simulink model "W06_city_highway_cs"  (R2019a)
settings: Solver=ode5  StartTime=0.0  StopTime=inf  FixedStep=1/60  RelTol=1e-3
PreLoadFcn:
  | mbxruntime.callbacks.PreLoadFcn(bdroot);
PostLoadFcn:
  | mbxruntime.callbacks.PostLoadFcn(bdroot);
InitFcn:
  | mbxruntime.callbacks.InitFcn(bdroot);
StartFcn:
  | mbxruntime.callbacks.StartFcn(bdroot);
StopFcn:
  | mbxruntime.callbacks.StopFcn(bdroot);
model workspace: external: MAT-File .\W06_city_highway_cs_hws.mat (data not in the file)
undefined symbols (not defined in the file or in its folder): DiscIntNeverNeededParam, FovAzimuth, FovAzimuthDefined, FovElevation, FovElevationDefined, Header, InitImageOutputDir, LocationX, LocationXDefined, LocationY, LocationYDefined, LocationZ, LocationZDefined, Orientation, OrientationPitch, OrientationPitchDefined, OrientationRoll, OrientationRollDefined, OrientationYaw, OrientationYawDefined, Poses, Poses_SL_Info, Position, W06_city_highway_cs_0270c22595f3b0e3, W06_city_highway_cs_086892688dd32ddc, W06_city_highway_cs_328c49ac39fca66b, W06_city_highway_cs_35ce05381b8ebe8c, W06_city_highway_cs_47b384f162638175, W06_city_highway_cs_766f76ce4de94dd5, W06_city_highway_cs_8c547f67cb81ffba, W06_city_highway_cs_aed52f2a7724a4f9, W06_city_highway_cs_Audi_A8_Sedan_1_Path_pathUniqueID, W06_city_highway_cs_b74cbb1f9f7331b5, W06_city_highway_cs_Citroen_C3_Hatchback_1_Path_pathUniqueID, W06_city_highway_cs_d395f8835e0c28b3, W06_city_highway_cs_e5f9d1759e19e2b4, W06_city_highway_cs_Toyota_Previa_MPV_1_Path_pathUniqueID
libraries: adeye_lib x26, simulink_extras x24, robotlib x7, sharedtransform x4, PreScanSimulinkLibrary x2, PreScanUsefulBlocks x1
(part 6 of 8)

== system W06_city_highway_cs/RoadsideLight_NL_2/Red_Mux ==
  MSCD [Cd] : Inport
  Position (xyz) [m] : Inport  Port=2
  Orientation (RPY) [deg] : Inport  Port=3
  Color [-] : Inport  Port=4
  TextureResourceID [-] : Inport  Port=5
  Bus Creator : BusCreator  Inputs='Intensity','Position','Orientation','Color','TextureResourceID'  OutDataTypeStr=Bus: PRESCAN_VISULIGHTACTUATOR_DATA  NonVirtualBus=on
  Bus Creator1 : BusCreator  Inputs=3  OutDataTypeStr=Bus: PRESCAN_RGB_DATA  NonVirtualBus=on
  Bus Creator2 : BusCreator  Inputs=3  OutDataTypeStr=Bus: PRESCAN_RPY_DATA  NonVirtualBus=on
  Bus Creator3 : BusCreator  Inputs=3  OutDataTypeStr=Bus: PRESCAN_XYZ_DATA  NonVirtualBus=on
  Data Type Conversion : DataTypeConversion  OutDataTypeStr=int32  RndMeth=Nearest
  Degrees to Radians : simulink_extras/Transformations/Degrees to Radians
  Demux : Demux  Outputs=3
  Demux1 : Demux  Outputs=3
  Demux2 : Demux  Outputs=3
  Lights : Outport
  wires:
  TextureResourceID [-]/1 -> Data Type Conversion/1  "TextureResourceID"
  MSCD [Cd]/1 -> Bus Creator/1  "Intensity"
  Bus Creator/1 -> Lights/1
  Demux/1 -> Bus Creator1/1  "R"
  Demux/2 -> Bus Creator1/2  "G"
  Demux/3 -> Bus Creator1/3  "B"
  Color [-]/1 -> Demux/1  "Color"
  Bus Creator1/1 -> Bus Creator/4  "Color"
  Demux1/1 -> Bus Creator2/1  "Roll"
  Demux1/2 -> Bus Creator2/2  "Pitch"
  Demux1/3 -> Bus Creator2/3  "Yaw"
  Orientation (RPY) [deg]/1 -> Degrees to Radians/1  "Orientation"
  Bus Creator2/1 -> Bus Creator/3  "Orientation"
  Demux2/1 -> Bus Creator3/1  "X"
  Demux2/2 -> Bus Creator3/2  "Y"
  Demux2/3 -> Bus Creator3/3  "Z"
  Position (xyz) [m]/1 -> Demux2/1  "Position"
  Bus Creator3/1 -> Bus Creator/2  "Position"
  Data Type Conversion/1 -> Bus Creator/5  "TextureResourceID"
  Degrees to Radians/1 -> Demux1/1

== system W06_city_highway_cs/RoadsideLight_NL_3/Green_Mux ==
  MSCD [Cd] : Inport
  Position (xyz) [m] : Inport  Port=2
  Orientation (RPY) [deg] : Inport  Port=3
  Color [-] : Inport  Port=4
  TextureResourceID [-] : Inport  Port=5
  Bus Creator : BusCreator  Inputs='Intensity','Position','Orientation','Color','TextureResourceID'  OutDataTypeStr=Bus: PRESCAN_VISULIGHTACTUATOR_DATA  NonVirtualBus=on
  Bus Creator1 : BusCreator  Inputs=3  OutDataTypeStr=Bus: PRESCAN_RGB_DATA  NonVirtualBus=on
  Bus Creator2 : BusCreator  Inputs=3  OutDataTypeStr=Bus: PRESCAN_RPY_DATA  NonVirtualBus=on
  Bus Creator3 : BusCreator  Inputs=3  OutDataTypeStr=Bus: PRESCAN_XYZ_DATA  NonVirtualBus=on
  Data Type Conversion : DataTypeConversion  OutDataTypeStr=int32  RndMeth=Nearest
  Degrees to Radians : simulink_extras/Transformations/Degrees to Radians
  Demux : Demux  Outputs=3
  Demux1 : Demux  Outputs=3
  Demux2 : Demux  Outputs=3
  Lights : Outport
  wires:
  TextureResourceID [-]/1 -> Data Type Conversion/1  "TextureResourceID"
  MSCD [Cd]/1 -> Bus Creator/1  "Intensity"
  Bus Creator/1 -> Lights/1
  Demux/1 -> Bus Creator1/1  "R"
  Demux/2 -> Bus Creator1/2  "G"
  Demux/3 -> Bus Creator1/3  "B"
  Color [-]/1 -> Demux/1  "Color"
  Bus Creator1/1 -> Bus Creator/4  "Color"
  Demux1/1 -> Bus Creator2/1  "Roll"
  Demux1/2 -> Bus Creator2/2  "Pitch"
  Demux1/3 -> Bus Creator2/3  "Yaw"
  Orientation (RPY) [deg]/1 -> Degrees to Radians/1  "Orientation"
  Bus Creator2/1 -> Bus Creator/3  "Orientation"
  Demux2/1 -> Bus Creator3/1  "X"
  Demux2/2 -> Bus Creator3/2  "Y"
  Demux2/3 -> Bus Creator3/3  "Z"
  Position (xyz) [m]/1 -> Demux2/1  "Position"
  Bus Creator3/1 -> Bus Creator/2  "Position"
  Data Type Conversion/1 -> Bus Creator/5  "TextureResourceID"
  Degrees to Radians/1 -> Demux1/1

== system W06_city_highway_cs/RoadsideLight_NL_3/Orange_Mux ==
  MSCD [Cd] : Inport
  Position (xyz) [m] : Inport  Port=2
  Orientation (RPY) [deg] : Inport  Port=3
  Color [-] : Inport  Port=4
  TextureResourceID [-] : Inport  Port=5
  Bus Creator : BusCreator  Inputs='Intensity','Position','Orientation','Color','TextureResourceID'  OutDataTypeStr=Bus: PRESCAN_VISULIGHTACTUATOR_DATA  NonVirtualBus=on
  Bus Creator1 : BusCreator  Inputs=3  OutDataTypeStr=Bus: PRESCAN_RGB_DATA  NonVirtualBus=on
  Bus Creator2 : BusCreator  Inputs=3  OutDataTypeStr=Bus: PRESCAN_RPY_DATA  NonVirtualBus=on
  Bus Creator3 : BusCreator  Inputs=3  OutDataTypeStr=Bus: PRESCAN_XYZ_DATA  NonVirtualBus=on
  Data Type Conversion : DataTypeConversion  OutDataTypeStr=int32  RndMeth=Nearest
  Degrees to Radians : simulink_extras/Transformations/Degrees to Radians
  Demux : Demux  Outputs=3
  Demux1 : Demux  Outputs=3
  Demux2 : Demux  Outputs=3
  Lights : Outport
  wires:
  TextureResourceID [-]/1 -> Data Type Conversion/1  "TextureResourceID"
  MSCD [Cd]/1 -> Bus Creator/1  "Intensity"
  Bus Creator/1 -> Lights/1
  Demux/1 -> Bus Creator1/1  "R"
  Demux/2 -> Bus Creator1/2  "G"
  Demux/3 -> Bus Creator1/3  "B"
  Color [-]/1 -> Demux/1  "Color"
  Bus Creator1/1 -> Bus Creator/4  "Color"
  Demux1/1 -> Bus Creator2/1  "Roll"
  Demux1/2 -> Bus Creator2/2  "Pitch"
  Demux1/3 -> Bus Creator2/3  "Yaw"
  Orientation (RPY) [deg]/1 -> Degrees to Radians/1  "Orientation"
  Bus Creator2/1 -> Bus Creator/3  "Orientation"
  Demux2/1 -> Bus Creator3/1  "X"
  Demux2/2 -> Bus Creator3/2  "Y"
  Demux2/3 -> Bus Creator3/3  "Z"
  Position (xyz) [m]/1 -> Demux2/1  "Position"
  Bus Creator3/1 -> Bus Creator/2  "Position"
  Data Type Conversion/1 -> Bus Creator/5  "TextureResourceID"
  Degrees to Radians/1 -> Demux1/1

== system W06_city_highway_cs/RoadsideLight_NL_3/Red_Mux ==
  MSCD [Cd] : Inport
  Position (xyz) [m] : Inport  Port=2
  Orientation (RPY) [deg] : Inport  Port=3
  Color [-] : Inport  Port=4
  TextureResourceID [-] : Inport  Port=5
  Bus Creator : BusCreator  Inputs='Intensity','Position','Orientation','Color','TextureResourceID'  OutDataTypeStr=Bus: PRESCAN_VISULIGHTACTUATOR_DATA  NonVirtualBus=on
  Bus Creator1 : BusCreator  Inputs=3  OutDataTypeStr=Bus: PRESCAN_RGB_DATA  NonVirtualBus=on
  Bus Creator2 : BusCreator  Inputs=3  OutDataTypeStr=Bus: PRESCAN_RPY_DATA  NonVirtualBus=on
  Bus Creator3 : BusCreator  Inputs=3  OutDataTypeStr=Bus: PRESCAN_XYZ_DATA  NonVirtualBus=on
  Data Type Conversion : DataTypeConversion  OutDataTypeStr=int32  RndMeth=Nearest
  Degrees to Radians : simulink_extras/Transformations/Degrees to Radians
  Demux : Demux  Outputs=3
  Demux1 : Demux  Outputs=3
  Demux2 : Demux  Outputs=3
  Lights : Outport
  wires:
  TextureResourceID [-]/1 -> Data Type Conversion/1  "TextureResourceID"
  MSCD [Cd]/1 -> Bus Creator/1  "Intensity"
  Bus Creator/1 -> Lights/1
  Demux/1 -> Bus Creator1/1  "R"
  Demux/2 -> Bus Creator1/2  "G"
  Demux/3 -> Bus Creator1/3  "B"
  Color [-]/1 -> Demux/1  "Color"
  Bus Creator1/1 -> Bus Creator/4  "Color"
  Demux1/1 -> Bus Creator2/1  "Roll"
  Demux1/2 -> Bus Creator2/2  "Pitch"
  Demux1/3 -> Bus Creator2/3  "Yaw"
  Orientation (RPY) [deg]/1 -> Degrees to Radians/1  "Orientation"
  Bus Creator2/1 -> Bus Creator/3  "Orientation"
  Demux2/1 -> Bus Creator3/1  "X"
  Demux2/2 -> Bus Creator3/2  "Y"
  Demux2/3 -> Bus Creator3/3  "Z"
  Position (xyz) [m]/1 -> Demux2/1  "Position"
  Bus Creator3/1 -> Bus Creator/2  "Position"
  Data Type Conversion/1 -> Bus Creator/5  "TextureResourceID"
  Degrees to Radians/1 -> Demux1/1

== system W06_city_highway_cs/RoadsideLight_NL_4/Green_Mux ==
  MSCD [Cd] : Inport
  Position (xyz) [m] : Inport  Port=2
  Orientation (RPY) [deg] : Inport  Port=3
  Color [-] : Inport  Port=4
  TextureResourceID [-] : Inport  Port=5
  Bus Creator : BusCreator  Inputs='Intensity','Position','Orientation','Color','TextureResourceID'  OutDataTypeStr=Bus: PRESCAN_VISULIGHTACTUATOR_DATA  NonVirtualBus=on
  Bus Creator1 : BusCreator  Inputs=3  OutDataTypeStr=Bus: PRESCAN_RGB_DATA  NonVirtualBus=on
  Bus Creator2 : BusCreator  Inputs=3  OutDataTypeStr=Bus: PRESCAN_RPY_DATA  NonVirtualBus=on
  Bus Creator3 : BusCreator  Inputs=3  OutDataTypeStr=Bus: PRESCAN_XYZ_DATA  NonVirtualBus=on
  Data Type Conversion : DataTypeConversion  OutDataTypeStr=int32  RndMeth=Nearest
  Degrees to Radians : simulink_extras/Transformations/Degrees to Radians
  Demux : Demux  Outputs=3
  Demux1 : Demux  Outputs=3
  Demux2 : Demux  Outputs=3
  Lights : Outport
  wires:
  TextureResourceID [-]/1 -> Data Type Conversion/1  "TextureResourceID"
  MSCD [Cd]/1 -> Bus Creator/1  "Intensity"
  Bus Creator/1 -> Lights/1
  Demux/1 -> Bus Creator1/1  "R"
  Demux/2 -> Bus Creator1/2  "G"
  Demux/3 -> Bus Creator1/3  "B"
  Color [-]/1 -> Demux/1  "Color"
  Bus Creator1/1 -> Bus Creator/4  "Color"
  Demux1/1 -> Bus Creator2/1  "Roll"
  Demux1/2 -> Bus Creator2/2  "Pitch"
  Demux1/3 -> Bus Creator2/3  "Yaw"
  Orientation (RPY) [deg]/1 -> Degrees to Radians/1  "Orientation"
  Bus Creator2/1 -> Bus Creator/3  "Orientation"
  Demux2/1 -> Bus Creator3/1  "X"
  Demux2/2 -> Bus Creator3/2  "Y"
  Demux2/3 -> Bus Creator3/3  "Z"
  Position (xyz) [m]/1 -> Demux2/1  "Position"
  Bus Creator3/1 -> Bus Creator/2  "Position"
  Data Type Conversion/1 -> Bus Creator/5  "TextureResourceID"
  Degrees to Radians/1 -> Demux1/1

== system W06_city_highway_cs/RoadsideLight_NL_4/Orange_Mux ==
  MSCD [Cd] : Inport
  Position (xyz) [m] : Inport  Port=2
  Orientation (RPY) [deg] : Inport  Port=3
  Color [-] : Inport  Port=4
  TextureResourceID [-] : Inport  Port=5
  Bus Creator : BusCreator  Inputs='Intensity','Position','Orientation','Color','TextureResourceID'  OutDataTypeStr=Bus: PRESCAN_VISULIGHTACTUATOR_DATA  NonVirtualBus=on
  Bus Creator1 : BusCreator  Inputs=3  OutDataTypeStr=Bus: PRESCAN_RGB_DATA  NonVirtualBus=on
  Bus Creator2 : BusCreator  Inputs=3  OutDataTypeStr=Bus: PRESCAN_RPY_DATA  NonVirtualBus=on
  Bus Creator3 : BusCreator  Inputs=3  OutDataTypeStr=Bus: PRESCAN_XYZ_DATA  NonVirtualBus=on
  Data Type Conversion : DataTypeConversion  OutDataTypeStr=int32  RndMeth=Nearest
  Degrees to Radians : simulink_extras/Transformations/Degrees to Radians
  Demux : Demux  Outputs=3
  Demux1 : Demux  Outputs=3
  Demux2 : Demux  Outputs=3
  Lights : Outport
  wires:
  TextureResourceID [-]/1 -> Data Type Conversion/1  "TextureResourceID"
  MSCD [Cd]/1 -> Bus Creator/1  "Intensity"
  Bus Creator/1 -> Lights/1
  Demux/1 -> Bus Creator1/1  "R"
  Demux/2 -> Bus Creator1/2  "G"
  Demux/3 -> Bus Creator1/3  "B"
  Color [-]/1 -> Demux/1  "Color"
  Bus Creator1/1 -> Bus Creator/4  "Color"
  Demux1/1 -> Bus Creator2/1  "Roll"
  Demux1/2 -> Bus Creator2/2  "Pitch"
  Demux1/3 -> Bus Creator2/3  "Yaw"
  Orientation (RPY) [deg]/1 -> Degrees to Radians/1  "Orientation"
  Bus Creator2/1 -> Bus Creator/3  "Orientation"
  Demux2/1 -> Bus Creator3/1  "X"
  Demux2/2 -> Bus Creator3/2  "Y"
  Demux2/3 -> Bus Creator3/3  "Z"
  Position (xyz) [m]/1 -> Demux2/1  "Position"
  Bus Creator3/1 -> Bus Creator/2  "Position"
  Data Type Conversion/1 -> Bus Creator/5  "TextureResourceID"
  Degrees to Radians/1 -> Demux1/1

== system W06_city_highway_cs/RoadsideLight_NL_4/Red_Mux ==
  MSCD [Cd] : Inport
  Position (xyz) [m] : Inport  Port=2
  Orientation (RPY) [deg] : Inport  Port=3
  Color [-] : Inport  Port=4
  TextureResourceID [-] : Inport  Port=5
  Bus Creator : BusCreator  Inputs='Intensity','Position','Orientation','Color','TextureResourceID'  OutDataTypeStr=Bus: PRESCAN_VISULIGHTACTUATOR_DATA  NonVirtualBus=on
  Bus Creator1 : BusCreator  Inputs=3  OutDataTypeStr=Bus: PRESCAN_RGB_DATA  NonVirtualBus=on
  Bus Creator2 : BusCreator  Inputs=3  OutDataTypeStr=Bus: PRESCAN_RPY_DATA  NonVirtualBus=on
  Bus Creator3 : BusCreator  Inputs=3  OutDataTypeStr=Bus: PRESCAN_XYZ_DATA  NonVirtualBus=on
  Data Type Conversion : DataTypeConversion  OutDataTypeStr=int32  RndMeth=Nearest
  Degrees to Radians : simulink_extras/Transformations/Degrees to Radians
  Demux : Demux  Outputs=3
  Demux1 : Demux  Outputs=3
  Demux2 : Demux  Outputs=3
  Lights : Outport
  wires:
  TextureResourceID [-]/1 -> Data Type Conversion/1  "TextureResourceID"
  MSCD [Cd]/1 -> Bus Creator/1  "Intensity"
  Bus Creator/1 -> Lights/1
  Demux/1 -> Bus Creator1/1  "R"
  Demux/2 -> Bus Creator1/2  "G"
  Demux/3 -> Bus Creator1/3  "B"
  Color [-]/1 -> Demux/1  "Color"
  Bus Creator1/1 -> Bus Creator/4  "Color"
  Demux1/1 -> Bus Creator2/1  "Roll"
  Demux1/2 -> Bus Creator2/2  "Pitch"
  Demux1/3 -> Bus Creator2/3  "Yaw"
  Orientation (RPY) [deg]/1 -> Degrees to Radians/1  "Orientation"
  Bus Creator2/1 -> Bus Creator/3  "Orientation"
  Demux2/1 -> Bus Creator3/1  "X"
  Demux2/2 -> Bus Creator3/2  "Y"
  Demux2/3 -> Bus Creator3/3  "Z"
  Position (xyz) [m]/1 -> Demux2/1  "Position"
  Bus Creator3/1 -> Bus Creator/2  "Position"
  Data Type Conversion/1 -> Bus Creator/5  "TextureResourceID"
  Degrees to Radians/1 -> Demux1/1

== system W06_city_highway_cs/Toyota_Previa_MPV_1/Car_Pos_and_Orient ==
  In1 : Inport
  In2 : Inport  Port=2
  In3 : Inport  Port=3
  In4 : Inport  Port=4
  In5 : Inport  Port=5
  In6 : Inport  Port=6
  Data Type Conversion : DataTypeConversion
  Data Type Conversion1 : DataTypeConversion
  Data Type Conversion2 : DataTypeConversion
  Degrees to Radians1 : simulink_extras/Transformations/Degrees to Radians
  Degrees to Radians2 : simulink_extras/Transformations/Degrees to Radians
  Degrees to Radians5 : simulink_extras/Transformations/Degrees to Radians
  Mux : Mux
  Rotation Angles to Quaternions : sharedtransform/Rotation Angles to Quaternions  rotationOrder=XYZ  aMode=aMode
      settings: SourceProductName=Aerospace Blockset  SourceProductBaseCode=AE
  Vector Concatenate2 : Concatenate  NumInputs=3
  Out1 : Outport
  wires:
  Degrees to Radians1/1 -> Vector Concatenate2/2
  Degrees to Radians5/1 -> Vector Concatenate2/1
  Vector Concatenate2/1 -> Rotation Angles to Quaternions/1
  Degrees to Radians2/1 -> Vector Concatenate2/3
  In1/1 -> Data Type Conversion/1
  In2/1 -> Data Type Conversion1/1
  In3/1 -> Data Type Conversion2/1
  In4/1 -> Degrees to Radians5/1
  In5/1 -> Degrees to Radians1/1
  In6/1 -> Degrees to Radians2/1
  Data Type Conversion/1 -> Mux/1
  Data Type Conversion1/1 -> Mux/2
  Data Type Conversion2/1 -> Mux/3
  Rotation Angles to Quaternions/1 -> Mux/4
  Mux/1 -> Out1/1

== system W06_city_highway_cs/Toyota_Previa_MPV_1/SELF_Demux ==
  SELF : Inport  OutDataTypeStr=Bus: PRESCAN_SELFSENSORDATA
  Bus Selector : BusSelector  OutputSignals=PositionX,PositionY,PositionZ,OrientationRoll,OrientationPitch,OrientationYaw,Velocity,Yaw_rate,Lat,Long,Alt
  Demux2 : Demux  Outputs=3
  Gain : Gain  Gain=180/pi
  Gain1 : Gain  Gain=180/pi
  Vector Concatenate1 : Concatenate  NumInputs=3
  compas converter : Subsystem
  x [m] : Outport
  y [m] : Outport  Port=2
  z [m] : Outport  Port=3
  rotx [deg] : Outport  Port=4
  roty [deg] : Outport  Port=5
  rotz [deg] : Outport  Port=6
  GPS lat [deg] : Outport  Port=7
  GPS long [deg] : Outport  Port=8
  GPS alt [m] : Outport  Port=9
  velocity [m/s] : Outport  Port=10
  heading [deg] : Outport  Port=11
  yaw rate [deg/s] : Outport  Port=12
  wires:
  Bus Selector/11 -> GPS alt [m]/1  "<Alt>"
  Bus Selector/10 -> GPS long [deg]/1  "<Long>"
  Bus Selector/9 -> GPS lat [deg]/1  "<Lat>"
  Bus Selector/8 -> Gain1/1  "<Yaw_rate>"
  Bus Selector/7 -> velocity [m/s]/1  "<Velocity>"
  Bus Selector/6 -> compas converter/1(rotz [rad]), Vector Concatenate1/3  "<OrientationYaw>"
  Bus Selector/5 -> Vector Concatenate1/2  "<OrientationPitch>"
  Bus Selector/4 -> Vector Concatenate1/1  "<OrientationRoll>"
  Vector Concatenate1/1 -> Gain/1
  Bus Selector/3 -> z [m]/1  "<PositionZ>"
  Bus Selector/2 -> y [m]/1  "<PositionY>"
  Bus Selector/1 -> x [m]/1  "<PositionX>"
  SELF/1 -> Bus Selector/1
  Gain/1 -> Demux2/1
  Demux2/1 -> rotx [deg]/1
  Demux2/2 -> roty [deg]/1
  Demux2/3 -> rotz [deg]/1
  compas converter/1(heading [deg]) -> heading [deg]/1
  Gain1/1 -> yaw rate [deg/s]/1

== system W06_city_highway_cs/Toyota_Previa_MPV_1/message_creator ==
  In1 : Inport
  Blank Message4 : robotlib/Blank Message  messageClass=Message  entityType=geometry_msgs/Pose  messageType=geometry_msgs/Pose  SampleTime=inf
      settings: SourceProductBaseCode=RO
  Bus Assignment3 : BusAssignment  AssignedSignals=Position.X,Position.Y,Position.Z,Orientation.W,Orientation.X,Orientation.Y,Orientation.Z
  Demux : Demux  Outputs=7
  Out1 : Outport
  wires:
  Blank Message4/1 -> Bus Assignment3/1
  Demux/4 -> Bus Assignment3/5
  Demux/3 -> Bus Assignment3/4
  Demux/5 -> Bus Assignment3/6
  Demux/7 -> Bus Assignment3/8
  Demux/2 -> Bus Assignment3/3
  In1/1 -> Demux/1
  Demux/6 -> Bus Assignment3/7
  Demux/1 -> Bus Assignment3/2
  Bus Assignment3/1 -> Out1/1

== system W06_city_highway_cs/Audi_A8_Sedan_1/SELF_Demux/compas converter ==
  rotz [rad] : Inport
  cart2compas : Subsystem
  rad2deg : Gain  Gain=180/pi
  heading [deg] : Outport
  wires:
  rad2deg/1 -> cart2compas/1(Angle [deg])
  rotz [rad]/1 -> rad2deg/1
  cart2compas/1(heading [deg]) -> heading [deg]/1

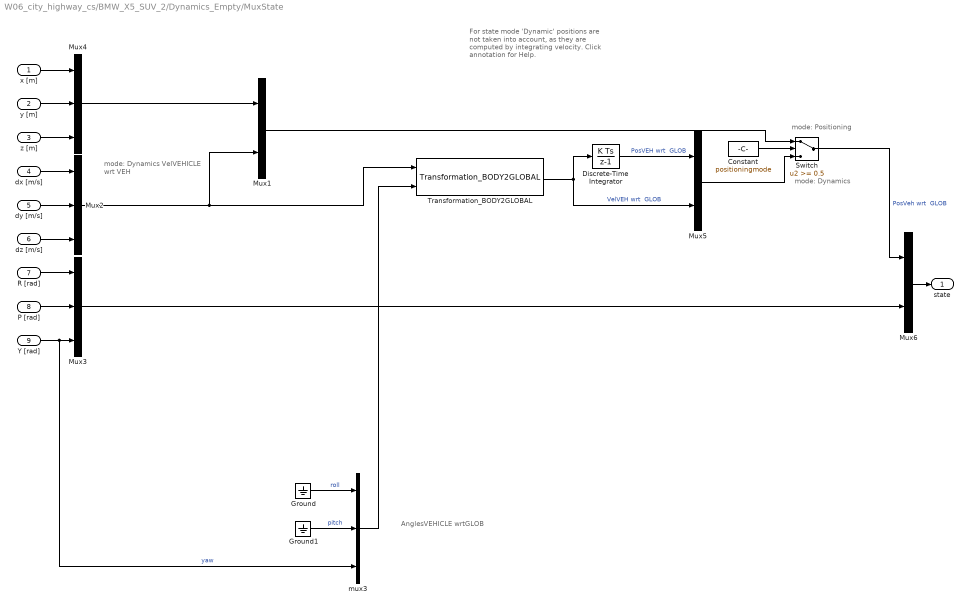
== system W06_city_highway_cs/BMW_X5_SUV_2/Dynamics_Empty/MuxState ==
  note: mode: Dynamics
  note: mode: Positioning
  note: mode: Dynamics
      | VelVEHICLE
      | wrt VEH
  note: AnglesVEHICLE
      | wrtGLOB
  note: For state mode 'Dynamic' positions
      | are not taken into account, as they
      | are computed by integrating velocity.
      | Click annotation for Help.
  x [m] : Inport  SampleTime=TimeStep
  y [m] : Inport  Port=2  SampleTime=TimeStep
  z [m] : Inport  Port=3  SampleTime=TimeStep
  dx [m/s] : Inport  Port=4  SampleTime=TimeStep
  dy [m/s] : Inport  Port=5  SampleTime=TimeStep
  dz [m/s] : Inport  Port=6  SampleTime=TimeStep
  R [rad] : Inport  Port=7  SampleTime=TimeStep
  P [rad] : Inport  Port=8  SampleTime=TimeStep
  Y [rad] : Inport  Port=9  SampleTime=TimeStep
  Constant : Constant  DisableCoverage=on  Value=positioningmode
  Discrete-Time Integrator : DiscreteIntegrator  SampleTime=TimeStep  ICPrevOutput=DiscIntNeverNeededParam  ICPrevScaledInput=DiscIntNeverNeededParam
  Ground : Ground
  Ground1 : Ground
  Mux1 : Mux  Inputs=[3 3]
  Mux2 : Mux  Inputs=3
  Mux3 : Mux  Inputs=3
  Mux4 : Mux  Inputs=3
  Mux5 : Mux  Inputs=[3 3]
  Mux6 : Mux  Inputs=[6 3]
  Switch : Switch  Threshold=0.5
  Transformation_BODY2GLOBAL : PreScanSimulinkLibrary/Simple_Vehicle_Dynamics/Chassis/MuxDynState/Transformation_BODY2GLOBAL  SystemSampleTime=-1
  mux3 : Mux  Inputs=3
  state : Outport
  wires:
  Constant/1 -> Switch/2
  Mux6/1 -> state/1
  Mux4/1 -> Mux1/1
  Mux5/1 -> Switch/3
  Mux1/1 -> Switch/1
  Switch/1 -> Mux6/1  "PosVeh wrt  GLOB"
  P [rad]/1 -> Mux3/2
  R [rad]/1 -> Mux3/1
  dz [m/s]/1 -> Mux2/3
  dy [m/s]/1 -> Mux2/2
  dx [m/s]/1 -> Mux2/1
  z [m]/1 -> Mux4/3
  y [m]/1 -> Mux4/2
  x [m]/1 -> Mux4/1
  Ground1/1 -> mux3/2  "pitch"
  Y [rad]/1 -> mux3/3, Mux3/3  "yaw"
  Mux3/1 -> Mux6/2
  Transformation_BODY2GLOBAL/1 -> Discrete-Time Integrator/1, Mux5/2  "VelVEH wrt  GLOB"
  mux3/1 -> Transformation_BODY2GLOBAL/2
  Ground/1 -> mux3/1  "roll"
  Mux2/1 -> Mux1/2, Transformation_BODY2GLOBAL/1
  Discrete-Time Integrator/1 -> Mux5/1  "PosVEH wrt  GLOB"

== system W06_city_highway_cs/BMW_X5_SUV_2/Dynamics_Empty/STATE_BMW_X5_SUV_2 ==
  State : Inport  SampleTime=TimeStep
  Bus Creator : BusCreator  Inputs=15  OutDataTypeStr=Bus: PRESCAN_STATEACTUATORDATA  NonVirtualBus=on
  Constant : Constant  Value=0
  Demux : Demux  Outputs=15
  Mux : Mux  Inputs=3
  Mux1 : Mux  Inputs=3
  Mux2 : Mux  Inputs=3
  iniBODYAngles wrtVEH [rad] : Constant  Value=Roll0  SampleTime=TimeStep
  iniBODYAngles wrtVEH [rad]1 : Constant  Value=Pitch0  SampleTime=TimeStep
  iniVEHAngles wrtGLOB [rad] : Constant  Value=Yaw0  SampleTime=TimeStep
  iniVEHposition wrtGLOB [m] : Constant  Value=x0  SampleTime=TimeStep
  iniVEHposition wrtGLOB [m]1 : Constant  Value=y0  SampleTime=TimeStep
  iniVEHposition wrtGLOB [m]2 : Constant  Value=z0  SampleTime=TimeStep
  state2FullState : PreScanSimulinkLibrary/state2FullState  SystemSampleTime=-1
  StateBus : Outport  OutDataTypeStr=Bus: PRESCAN_STATEACTUATORDATA
  wires:
  Mux2/1 -> state2FullState/4
  iniVEHAngles wrtGLOB [rad]/1 -> Mux2/3
  Mux1/1 -> state2FullState/3
  Constant/1 -> Mux2/1, Mux2/2, Mux1/3
  iniBODYAngles wrtVEH [rad]1/1 -> Mux1/2
  iniBODYAngles wrtVEH [rad]/1 -> Mux1/1
  Mux/1 -> state2FullState/2
  iniVEHposition wrtGLOB [m]2/1 -> Mux/3
  iniVEHposition wrtGLOB [m]/1 -> Mux/1
  iniVEHposition wrtGLOB [m]1/1 -> Mux/2
  Demux/15 -> Bus Creator/15  "AngularVelocityYaw"
  Demux/14 -> Bus Creator/14  "AngularVelocityPitch"
  Demux/13 -> Bus Creator/13  "AngularVelocityRoll"
  Demux/12 -> Bus Creator/12  "OrientationYaw"
  Demux/11 -> Bus Creator/11  "OrientationPitch"
  Demux/10 -> Bus Creator/10  "OrientationRoll"
  Demux/9 -> Bus Creator/9  "AccelerationZ"
  Demux/8 -> Bus Creator/8  "AccelerationY"
  Demux/7 -> Bus Creator/7  "AccelerationX"
  Demux/6 -> Bus Creator/6  "VelocityZ"
  Demux/5 -> Bus Creator/5  "VelocityY"
  Demux/4 -> Bus Creator/4  "VelocityX"
  Demux/3 -> Bus Creator/3  "PositionZ"
  Demux/2 -> Bus Creator/2  "PositionY"
  Demux/1 -> Bus Creator/1  "PositionX"
  state2FullState/1 -> Demux/1
  State/1 -> state2FullState/1
  Bus Creator/1 -> StateBus/1

== system W06_city_highway_cs/BMW_X5_SUV_2/Dynamics_Empty/Subsystem ==
  note: Current
  note: Desired
  In1 : Inport
  In2 : Inport  Port=2
  Constant : Constant  Value=0.05
  If : If  NumInputs=2  IfExpression=u1 > u2  ElseIfExpressions=u1 > -u2
  If Action Subsystem : Subsystem  TreatAsAtomicUnit=on
  If Action Subsystem1 : Subsystem  TreatAsAtomicUnit=on
  If Action Subsystem2 : Subsystem  TreatAsAtomicUnit=on
  Merge : Merge  Inputs=3
  Subtract : Sum  Inputs=-+
  Out1 : Outport
  wires:
  Constant/1 -> If/2, If Action Subsystem/2(In2), If Action Subsystem1/2(In2)
  Subtract/1 -> If/1
  In2/1 -> If Action Subsystem2/1(In1), Subtract/2
  In1/1 -> Subtract/1, If Action Subsystem/1(In1), If Action Subsystem1/1(In1)
  If Action Subsystem1/1(Out1) -> Merge/3
  If/1 -> If Action Subsystem/Action
  If/2 -> If Action Subsystem2/Action
  If Action Subsystem2/1(Out1) -> Merge/2
  Merge/1 -> Out1/1
  If/3 -> If Action Subsystem1/Action
  If Action Subsystem/1(Out1) -> Merge/1

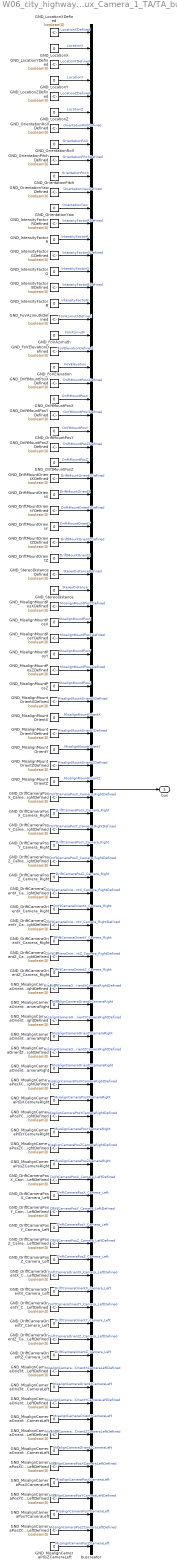
== system W06_city_highway_cs/BMW_X5_SUV_2/Mux_Camera_1_TA/TA_bus ==
  GND_DriftCameraOrientX_Camera_Left : Constant  Value=0
  GND_DriftCameraOrientX_Camera_LeftDefined : Constant  Value=boolean(0)
  GND_DriftCameraOrientX_Camera_Right : Constant  Value=0
  GND_DriftCameraOrientX_Camera_RightDefined : Constant  Value=boolean(0)
  GND_DriftCameraOrientY_Camera_Left : Constant  Value=0
  GND_DriftCameraOrientY_Camera_LeftDefined : Constant  Value=boolean(0)
  GND_DriftCameraOrientY_Camera_Right : Constant  Value=0
  GND_DriftCameraOrientY_Camera_RightDefined : Constant  Value=boolean(0)
  GND_DriftCameraOrientZ_Camera_Left : Constant  Value=0
  GND_DriftCameraOrientZ_Camera_LeftDefined : Constant  Value=boolean(0)
  GND_DriftCameraOrientZ_Camera_Right : Constant  Value=0
  GND_DriftCameraOrientZ_Camera_RightDefined : Constant  Value=boolean(0)
  GND_DriftCameraPosX_Camera_Left : Constant  Value=0
  GND_DriftCameraPosX_Camera_LeftDefined : Constant  Value=boolean(0)
  GND_DriftCameraPosX_Camera_Right : Constant  Value=0
  GND_DriftCameraPosX_Camera_RightDefined : Constant  Value=boolean(0)
  GND_DriftCameraPosY_Camera_Left : Constant  Value=0
  GND_DriftCameraPosY_Camera_LeftDefined : Constant  Value=boolean(0)
  GND_DriftCameraPosY_Camera_Right : Constant  Value=0
  GND_DriftCameraPosY_Camera_RightDefined : Constant  Value=boolean(0)
  GND_DriftCameraPosZ_Camera_Left : Constant  Value=0
  GND_DriftCameraPosZ_Camera_LeftDefined : Constant  Value=boolean(0)
  GND_DriftCameraPosZ_Camera_Right : Constant  Value=0
  GND_DriftCameraPosZ_Camera_RightDefined : Constant  Value=boolean(0)
  GND_DriftMountOrientX : Constant  Value=0
  GND_DriftMountOrientXDefined : Constant  Value=boolean(0)
  GND_DriftMountOrientY : Constant  Value=0
  GND_DriftMountOrientYDefined : Constant  Value=boolean(0)
  GND_DriftMountOrientZ : Constant  Value=0
  GND_DriftMountOrientZDefined : Constant  Value=boolean(0)
  GND_DriftMountPosX : Constant  Value=0
  GND_DriftMountPosXDefined : Constant  Value=boolean(0)
  GND_DriftMountPosY : Constant  Value=0
  GND_DriftMountPosYDefined : Constant  Value=boolean(0)
  GND_DriftMountPosZ : Constant  Value=0
  GND_DriftMountPosZDefined : Constant  Value=boolean(0)
  GND_FoVAzimuth : Constant  Value=0
  GND_FoVAzimuthDefined : Constant  Value=boolean(0)
  GND_FoVElevation : Constant  Value=0
  GND_FoVElevationDefined : Constant  Value=boolean(0)
  GND_IntensityFactorB : Constant  Value=0
  GND_IntensityFactorBDefined : Constant  Value=boolean(0)
  GND_IntensityFactorG : Constant  Value=0
  GND_IntensityFactorGDefined : Constant  Value=boolean(0)
  GND_IntensityFactorR : Constant  Value=0
  GND_IntensityFactorRDefined : Constant  Value=boolean(0)
  GND_LocationX : Constant  Value=0
  GND_LocationXDefined : Constant  Value=boolean(0)
  GND_LocationY : Constant  Value=0
  GND_LocationYDefined : Constant  Value=boolean(0)
  GND_LocationZ : Constant  Value=0
  GND_LocationZDefined : Constant  Value=boolean(0)
  GND_MisalignCameraOrientXCameraLeft : Constant  Value=0
  GND_MisalignCameraOrientXCameraLeftDefined : Constant  Value=boolean(0)
  GND_MisalignCameraOrientXCameraRight : Constant  Value=0
  GND_MisalignCameraOrientXCameraRightDefined : Constant  Value=boolean(0)
  GND_MisalignCameraOrientYCameraLeft : Constant  Value=0
  GND_MisalignCameraOrientYCameraLeftDefined : Constant  Value=boolean(0)
  GND_MisalignCameraOrientYCameraRight : Constant  Value=0
  GND_MisalignCameraOrientYCameraRightDefined : Constant  Value=boolean(0)
  GND_MisalignCameraOrientZCameraLeft : Constant  Value=0
  GND_MisalignCameraOrientZCameraLeftDefined : Constant  Value=boolean(0)
  GND_MisalignCameraOrientZCameraRight : Constant  Value=0
  GND_MisalignCameraOrientZCameraRightDefined : Constant  Value=boolean(0)
  GND_MisalignCameraPosXCameraLeft : Constant  Value=0
  GND_MisalignCameraPosXCameraLeftDefined : Constant  Value=boolean(0)
  GND_MisalignCameraPosXCameraRight : Constant  Value=0
  GND_MisalignCameraPosXCameraRightDefined : Constant  Value=boolean(0)
  GND_MisalignCameraPosYCameraLeft : Constant  Value=0
  GND_MisalignCameraPosYCameraLeftDefined : Constant  Value=boolean(0)
  GND_MisalignCameraPosYCameraRight : Constant  Value=0
  GND_MisalignCameraPosYCameraRightDefined : Constant  Value=boolean(0)
  GND_MisalignCameraPosZCameraLeft : Constant  Value=0
  GND_MisalignCameraPosZCameraLeftDefined : Constant  Value=boolean(0)
  GND_MisalignCameraPosZCameraRight : Constant  Value=0
  GND_MisalignCameraPosZCameraRightDefined : Constant  Value=boolean(0)
  GND_MisalignMountOrientX : Constant  Value=0
  GND_MisalignMountOrientXDefined : Constant  Value=boolean(0)
  GND_MisalignMountOrientY : Constant  Value=0
  GND_MisalignMountOrientYDefined : Constant  Value=boolean(0)
  GND_MisalignMountOrientZ : Constant  Value=0
  GND_MisalignMountOrientZDefined : Constant  Value=boolean(0)
  GND_MisalignMountPosX : Constant  Value=0
  GND_MisalignMountPosXDefined : Constant  Value=boolean(0)
  GND_MisalignMountPosY : Constant  Value=0
  GND_MisalignMountPosYDefined : Constant  Value=boolean(0)
  GND_MisalignMountPosZ : Constant  Value=0
  GND_MisalignMountPosZDefined : Constant  Value=boolean(0)
  GND_OrientationPitch : Constant  Value=0
  GND_OrientationPitchDefined : Constant  Value=boolean(0)
  GND_OrientationRoll : Constant  Value=0
  GND_OrientationRollDefined : Constant  Value=boolean(0)
  GND_OrientationYaw : Constant  Value=0
  GND_OrientationYawDefined : Constant  Value=boolean(0)
  GND_StereoDistance : Constant  Value=0
  GND_StereoDistanceDefined : Constant  Value=boolean(0)
  buscreator : BusCreator  Inputs=96  OutDataTypeStr=Bus: PRESCAN_CAMERASENSOR_TA  NonVirtualBus=on
  bus : Outport  OutDataTypeStr=Bus: PRESCAN_CAMERASENSOR_TA
  wires:
  GND_LocationXDefined/1 -> buscreator/1  "LocationXDefined"
  GND_LocationX/1 -> buscreator/2  "LocationX"
  GND_LocationYDefined/1 -> buscreator/3  "LocationYDefined"
  GND_LocationY/1 -> buscreator/4  "LocationY"
  GND_LocationZDefined/1 -> buscreator/5  "LocationZDefined"
  GND_LocationZ/1 -> buscreator/6  "LocationZ"
  GND_OrientationRollDefined/1 -> buscreator/7  "OrientationRollDefined"
  GND_OrientationRoll/1 -> buscreator/8  "OrientationRoll"
  GND_OrientationPitchDefined/1 -> buscreator/9  "OrientationPitchDefined"
  GND_OrientationPitch/1 -> buscreator/10  "OrientationPitch"
  GND_OrientationYawDefined/1 -> buscreator/11  "OrientationYawDefined"
  GND_OrientationYaw/1 -> buscreator/12  "OrientationYaw"
  GND_IntensityFactorRDefined/1 -> buscreator/13  "IntensityFactorRDefined"
  GND_IntensityFactorR/1 -> buscreator/14  "IntensityFactorR"
  GND_IntensityFactorGDefined/1 -> buscreator/15  "IntensityFactorGDefined"
  GND_IntensityFactorG/1 -> buscreator/16  "IntensityFactorG"
  GND_IntensityFactorBDefined/1 -> buscreator/17  "IntensityFactorBDefined"
  GND_IntensityFactorB/1 -> buscreator/18  "IntensityFactorB"
  GND_FoVAzimuthDefined/1 -> buscreator/19  "FoVAzimuthDefined"
  GND_FoVAzimuth/1 -> buscreator/20  "FoVAzimuth"
  GND_FoVElevationDefined/1 -> buscreator/21  "FoVElevationDefined"
  GND_FoVElevation/1 -> buscreator/22  "FoVElevation"
  GND_DriftMountPosXDefined/1 -> buscreator/23  "DriftMountPosXDefined"
  GND_DriftMountPosX/1 -> buscreator/24  "DriftMountPosX"
  GND_DriftMountPosYDefined/1 -> buscreator/25  "DriftMountPosYDefined"
  GND_DriftMountPosY/1 -> buscreator/26  "DriftMountPosY"
  GND_DriftMountPosZDefined/1 -> buscreator/27  "DriftMountPosZDefined"
  GND_DriftMountPosZ/1 -> buscreator/28  "DriftMountPosZ"
  GND_DriftMountOrientXDefined/1 -> buscreator/29  "DriftMountOrientXDefined"
  GND_DriftMountOrientX/1 -> buscreator/30  "DriftMountOrientX"
  GND_DriftMountOrientYDefined/1 -> buscreator/31  "DriftMountOrientYDefined"
  GND_DriftMountOrientY/1 -> buscreator/32  "DriftMountOrientY"
  GND_DriftMountOrientZDefined/1 -> buscreator/33  "DriftMountOrientZDefined"
  GND_DriftMountOrientZ/1 -> buscreator/34  "DriftMountOrientZ"
  GND_StereoDistanceDefined/1 -> buscreator/35  "StereoDistanceDefined"
  GND_StereoDistance/1 -> buscreator/36  "StereoDistance"
  GND_MisalignMountPosXDefined/1 -> buscreator/37  "MisalignMountPosXDefined"
  GND_MisalignMountPosX/1 -> buscreator/38  "MisalignMountPosX"
  GND_MisalignMountPosYDefined/1 -> buscreator/39  "MisalignMountPosYDefined"
  GND_MisalignMountPosY/1 -> buscreator/40  "MisalignMountPosY"
  GND_MisalignMountPosZDefined/1 -> buscreator/41  "MisalignMountPosZDefined"
  GND_MisalignMountPosZ/1 -> buscreator/42  "MisalignMountPosZ"
  GND_MisalignMountOrientXDefined/1 -> buscreator/43  "MisalignMountOrientXDefined"
  GND_MisalignMountOrientX/1 -> buscreator/44  "MisalignMountOrientX"
  GND_MisalignMountOrientYDefined/1 -> buscreator/45  "MisalignMountOrientYDefined"
  GND_MisalignMountOrientY/1 -> buscreator/46  "MisalignMountOrientY"
  GND_MisalignMountOrientZDefined/1 -> buscreator/47  "MisalignMountOrientZDefined"
  GND_MisalignMountOrientZ/1 -> buscreator/48  "MisalignMountOrientZ"
  GND_DriftCameraPosX_Camera_RightDefined/1 -> buscreator/49  "DriftCameraPosX_Camera_RightDefined"
  GND_DriftCameraPosX_Camera_Right/1 -> buscreator/50  "DriftCameraPosX_Camera_Right"
  GND_DriftCameraPosY_Camera_RightDefined/1 -> buscreator/51  "DriftCameraPosY_Camera_RightDefined"
  GND_DriftCameraPosY_Camera_Right/1 -> buscreator/52  "DriftCameraPosY_Camera_Right"
  GND_DriftCameraPosZ_Camera_RightDefined/1 -> buscreator/53  "DriftCameraPosZ_Camera_RightDefined"
  GND_DriftCameraPosZ_Camera_Right/1 -> buscreator/54  "DriftCameraPosZ_Camera_Right"
  GND_DriftCameraOrientX_Camera_RightDefined/1 -> buscreator/55  "DriftCameraOrientX_Camera_RightDefined"
  GND_DriftCameraOrientX_Camera_Right/1 -> buscreator/56  "DriftCameraOrientX_Camera_Right"
  GND_DriftCameraOrientY_Camera_RightDefined/1 -> buscreator/57  "DriftCameraOrientY_Camera_RightDefined"
  GND_DriftCameraOrientY_Camera_Right/1 -> buscreator/58  "DriftCameraOrientY_Camera_Right"
  GND_DriftCameraOrientZ_Camera_RightDefined/1 -> buscreator/59  "DriftCameraOrientZ_Camera_RightDefined"
  GND_DriftCameraOrientZ_Camera_Right/1 -> buscreator/60  "DriftCameraOrientZ_Camera_Right"
  GND_MisalignCameraOrientXCameraRightDefined/1 -> buscreator/61  "MisalignCameraOrientXCameraRightDefined"
  GND_MisalignCameraOrientXCameraRight/1 -> buscreator/62  "MisalignCameraOrientXCameraRight"
  GND_MisalignCameraOrientYCameraRightDefined/1 -> buscreator/63  "MisalignCameraOrientYCameraRightDefined"
  GND_MisalignCameraOrientYCameraRight/1 -> buscreator/64  "MisalignCameraOrientYCameraRight"
  GND_MisalignCameraOrientZCameraRightDefined/1 -> buscreator/65  "MisalignCameraOrientZCameraRightDefined"
  GND_MisalignCameraOrientZCameraRight/1 -> buscreator/66  "MisalignCameraOrientZCameraRight"
  GND_MisalignCameraPosXCameraRightDefined/1 -> buscreator/67  "MisalignCameraPosXCameraRightDefined"
  GND_MisalignCameraPosXCameraRight/1 -> buscreator/68  "MisalignCameraPosXCameraRight"
  GND_MisalignCameraPosYCameraRightDefined/1 -> buscreator/69  "MisalignCameraPosYCameraRightDefined"
  GND_MisalignCameraPosYCameraRight/1 -> buscreator/70  "MisalignCameraPosYCameraRight"
  GND_MisalignCameraPosZCameraRightDefined/1 -> buscreator/71  "MisalignCameraPosZCameraRightDefined"
  GND_MisalignCameraPosZCameraRight/1 -> buscreator/72  "MisalignCameraPosZCameraRight"
  GND_DriftCameraPosX_Camera_LeftDefined/1 -> buscreator/73  "DriftCameraPosX_Camera_LeftDefined"
  GND_DriftCameraPosX_Camera_Left/1 -> buscreator/74  "DriftCameraPosX_Camera_Left"
  GND_DriftCameraPosY_Camera_LeftDefined/1 -> buscreator/75  "DriftCameraPosY_Camera_LeftDefined"
  GND_DriftCameraPosY_Camera_Left/1 -> buscreator/76  "DriftCameraPosY_Camera_Left"
  GND_DriftCameraPosZ_Camera_LeftDefined/1 -> buscreator/77  "DriftCameraPosZ_Camera_LeftDefined"
  GND_DriftCameraPosZ_Camera_Left/1 -> buscreator/78  "DriftCameraPosZ_Camera_Left"
  GND_DriftCameraOrientX_Camera_LeftDefined/1 -> buscreator/79  "DriftCameraOrientX_Camera_LeftDefined"
  GND_DriftCameraOrientX_Camera_Left/1 -> buscreator/80  "DriftCameraOrientX_Camera_Left"
  GND_DriftCameraOrientY_Camera_LeftDefined/1 -> buscreator/81  "DriftCameraOrientY_Camera_LeftDefined"
  GND_DriftCameraOrientY_Camera_Left/1 -> buscreator/82  "DriftCameraOrientY_Camera_Left"
  GND_DriftCameraOrientZ_Camera_LeftDefined/1 -> buscreator/83  "DriftCameraOrientZ_Camera_LeftDefined"
  GND_DriftCameraOrientZ_Camera_Left/1 -> buscreator/84  "DriftCameraOrientZ_Camera_Left"
  GND_MisalignCameraOrientXCameraLeftDefined/1 -> buscreator/85  "MisalignCameraOrientXCameraLeftDefined"
  GND_MisalignCameraOrientXCameraLeft/1 -> buscreator/86  "MisalignCameraOrientXCameraLeft"
  GND_MisalignCameraOrientYCameraLeftDefined/1 -> buscreator/87  "MisalignCameraOrientYCameraLeftDefined"
  GND_MisalignCameraOrientYCameraLeft/1 -> buscreator/88  "MisalignCameraOrientYCameraLeft"
  GND_MisalignCameraOrientZCameraLeftDefined/1 -> buscreator/89  "MisalignCameraOrientZCameraLeftDefined"
  GND_MisalignCameraOrientZCameraLeft/1 -> buscreator/90  "MisalignCameraOrientZCameraLeft"
  GND_MisalignCameraPosXCameraLeftDefined/1 -> buscreator/91  "MisalignCameraPosXCameraLeftDefined"
  GND_MisalignCameraPosXCameraLeft/1 -> buscreator/92  "MisalignCameraPosXCameraLeft"
  GND_MisalignCameraPosYCameraLeftDefined/1 -> buscreator/93  "MisalignCameraPosYCameraLeftDefined"
  GND_MisalignCameraPosYCameraLeft/1 -> buscreator/94  "MisalignCameraPosYCameraLeft"
  GND_MisalignCameraPosZCameraLeftDefined/1 -> buscreator/95  "MisalignCameraPosZCameraLeftDefined"
  GND_MisalignCameraPosZCameraLeft/1 -> buscreator/96  "MisalignCameraPosZCameraLeft"
  buscreator/1 -> bus/1
